simulink model "TuningCommandGenerator"  (R2016b)
settings: Solver=FixedStepDiscrete  StartTime=0.0  StopTime=inf  RelTol=1e-3  EnableMultiTasking=on
settings Model: xpc_rtwmakecfg_data=_xpcethercatlib_  Creator=march  LastModifiedBy=march
settings SolverCC: EnableConcurrentExecution=on  AutoInsertRateTranBlk=on
settings DataIOCC: SaveFormat=StructureWithTime  SaveOutput=off  SaveTime=off
settings OptimizationCC: BlockReduction=off  OptimizeBlockIOStorage=off  BufferReuse=off  GlobalBufferReuse=off  ExpressionFolding=off  LocalBlockOutputs=off
settings HardwareCC: ProdBitPerPointer=32  ProdBitPerSizeT=32  ProdBitPerPtrDiffT=32  ProdLargestAtomicFloat=None  ProdWordSize=32  ProdLongLongMode=on  ProdHWDeviceType=Generic->32-bit x86 compatible
settings RTWCC: SystemTargetFile=slrt.tlc  TemplateMakefile=slrt_default_tmf  PostCodeGenCommand=SomanetTuning_make_rtw_hook  Description=Simulink Real-Time  RTWVerbose=off  CodeExecutionProfiling=on  RTWCompilerOptimization=on
settings SimulinkRealTimeCC: xPCModelTimeoutSecs=20

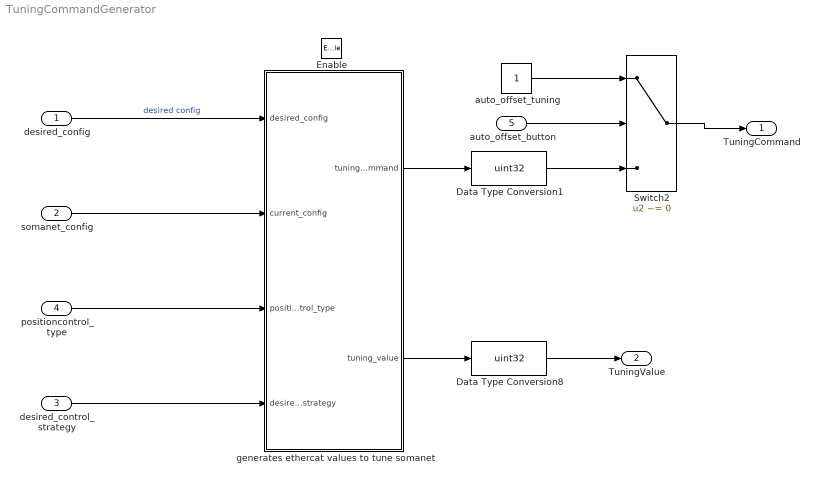
== system TuningCommandGenerator ==
  desired_config : Inport  OutDataTypeStr=int32  PortDimensions=15  SampleTime=0.002
  somanet_config : Inport  Port=2  OutDataTypeStr=double  PortDimensions=15  SampleTime=[0.002,0]
  desired_control_strategy : Inport  Port=3  OutDataTypeStr=int8  PortDimensions=1  SampleTime=0
  positioncontrol_type : Inport  Port=4  OutDataTypeStr=int32  PortDimensions=1  SampleTime=0.002
  auto_offset_button : Inport  Port=5  OutDataTypeStr=double  PortDimensions=1  SampleTime=0.002
  Enable : EnablePort  OutDataTypeStr=boolean
  Data Type Conversion1 : DataTypeConversion  OutDataTypeStr=uint32
  Data Type Conversion8 : DataTypeConversion  OutDataTypeStr=uint32
  Switch2 : Switch  Criteria=u2 ~= 0
  auto_offset_tuning : Constant  OutDataTypeStr=uint32
  generates ethercat values to tune somanet : MATLAB Function  TreatAsAtomicUnit=on  SystemSampleTime=0.002
  TuningCommand : Outport  OutDataTypeStr=uint32  PortDimensions=1  SampleTime=[0.002,0]
  TuningValue : Outport  Port=2  OutDataTypeStr=uint32  PortDimensions=1  SampleTime=[0.002,0]
  wires:
  positioncontrol_type/1 -> generates ethercat values to tune somanet/3(positioncontrol_type)
  Data Type Conversion8/1 -> TuningValue/1
  generates ethercat values to tune somanet/2(tuning_value) -> Data Type Conversion8/1
  desired_control_strategy/1 -> generates ethercat values to tune somanet/4(desired_control_strategy)
  desired_config/1 -> generates ethercat values to tune somanet/1(desired_config)  "desired config"
  somanet_config/1 -> generates ethercat values to tune somanet/2(current_config)
  auto_offset_button/1 -> Switch2/2
  generates ethercat values to tune somanet/1(tuning_command) -> Data Type Conversion1/1
  Data Type Conversion1/1 -> Switch2/3
  Switch2/1 -> TuningCommand/1
  auto_offset_tuning/1 -> Switch2/1

== matlab function TuningCommandGenerator/generates ethercat values to tune somanet ==
  data: desired_config input; current_config input; tuning_command output; positioncontrol_type input; tuning_value output; desired_control_strategy input
function [tuning_command,tuning_value] = gen_tuning_command(desired_config,current_config, positioncontrol_type ,desired_control_strategy)
    persistent lookup;
    persistent last_control_strategy;
    persistent last2_control_strategy;
    persistent last_positioncontrol_type;
    persistent has_issued_command;
    persistent command_timeout;
    
    if (isempty(lookup))
        lookup = [hex2dec('A0'),... %
        hex2dec('B0'),... %
        hex2dec('CC'),... %
        hex2dec('CB'),... %
        hex2dec('CA'),... %
        hex2dec('E0'),... % 
        hex2dec('C0') + 0,hex2dec('C0') + 1,hex2dec('C0') + 2,hex2dec('C0') + 3,... %
        hex2dec('C6') + 0,hex2dec('C6') + 1,hex2dec('C6') + 2,hex2dec('C6') + 3,... %
        hex2dec('CD')]; %
        last_control_strategy = int8(0);
        last2_control_strategy = int8(0);
        last_positioncontrol_type = int32(0);
        has_issued_command = false;
        command_timeout = 0;
    end
    
    if command_timeout > 0
        tuning_command = int32(0);
        tuning_value = int32(0);
        command_timeout = command_timeout -1;
        return;
    end
    
    if(has_issued_command)
        tuning_command = int32(0); %send Ack to Somanet, so it's ready for the next command
        tuning_value = int32(0);
        has_issued_command = false;
        command_timeout = 10; %% Wait 10 loops, which should be 10 * sampletime = 10 * 0.002 = 0.02
        return
    end
    
    for i=1:size(current_config,1)
        if current_config(i) ~= desired_config(i)
            tuning_command = int32(lookup(i));
            tuning_value = desired_config(i);
            has_issued_command = true;
            return;
        end
    end
    
    if last_control_strategy ~= last2_control_strategy
        last2_control_strategy = last_control_strategy;
        tuning_command = int32(0); %send Ack to Somanet, so it's ready for the next command
        tuning_value = int32(0);
        return;
    end
    
    if desired_control_strategy ~= last_control_strategy || positioncontrol_type ~= last_positioncontrol_type
        last_control_strategy = desired_control_strategy;
        if last_positioncontrol_type ~= positioncontrol_type
            last_positioncontrol_type = positioncontrol_type;
            last2_control_strategy = int8(0); % so an Ack will be sent next loop
        end
        disp(['Sending control command to tuning app: ', desired_control_strategy]);
        tuning_command = int32(desired_control_strategy); % these coincide, nice
        tuning_value = positioncontrol_type; % this value is not used when controlstrategy is not position, so this is fine 
        return;
    end    
    

    tuning_command = int32(0);
    tuning_value = int32(0);
end
